simulink model "ADCS_trainee0"  (R2020b)
settings: Solver=ode23t  StartTime=0.0  StopTime=250  RelTol=1e-4
values from neighbouring files (symbols this model uses):
  J = eye(3)*((massa_sat*((d^2)/6))+Jr)    [ADCS_main_trainee.m]
  Jr = 3e-6    (= 3e-06)    [ADCS_main_trainee.m]
  mag_ref = [2 -5 3]'    [ADCS_main_trainee.m]
  sol_ref = [5 -1 1]'    [ADCS_main_trainee.m]
  T = 5    [ADCS_main_trainee.m]
  vel_ang_inicial = [0 6e-2 0]'    [ADCS_main_trainee.m]
undefined symbols (not defined in the file or in its folder): b, Kiw, Km, Kpw
libraries: vrlib x4, aerolibutil x3, pid_lib x2, aerolibanim x1, sharedutil x1, sharedtransform x1
settings Model: Creator=felip  LastModifiedBy=elder
settings SolverCC: ZeroCrossAlgorithm=Adaptive  AutoInsertRateTranBlk=on
settings DebuggingCC: IgnoredZcDiagnostic=none

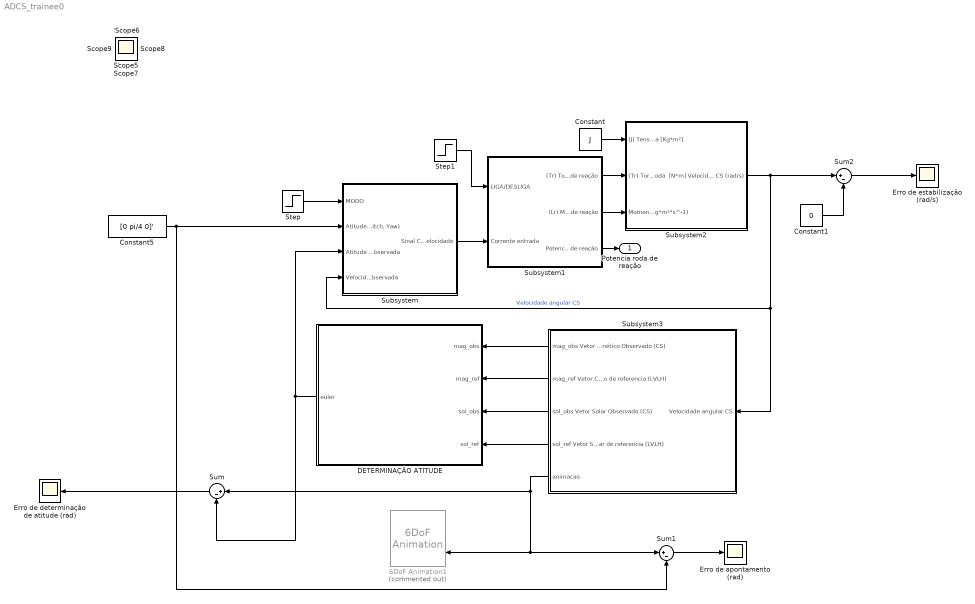
== system ADCS_trainee0 ==
  6DoF Animation1 : aerolibanim/6DoF Animation  Commented=on  u1=[-15 15 -15 15 -15 15]  u2=0.1  u3=0.81  u4=[0 0 0]  u5=Fly alongside  u6=[150 150 -150]  u7=10  u8=on
  Constant : Constant  Value=J
  Constant1 : Constant  Value=0
  Constant5 : Constant  Value=[0 pi/4 0]'
  DETERMINAÇÂO ATITUDE : MATLAB Function  TreatAsAtomicUnit=on  SystemSampleTime=1e-1
  Erro de apontamento (rad) : Scope
  Erro de determinação de atitude (rad) : Scope
  Erro de estabilização (rad/s) : Scope
  Step : Step  Time=130  Before=1  After=0  SampleTime=0
  Step1 : Step  Time=10  SampleTime=0
  Subsystem : Subsystem
      mask Display:
      | image('$imagefile'); % Use "Edit Image" on toolstrip to change.
      | 
      | port_label('input', 1, 'modo', 'texmode', 'on')
      | port_label('input', 2, 'ati_{des}', 'texmode', 'on')
      | port_label('input', 3, 'ati_{obs}', 'texmode', 'on')
      | port_label('input', 4, '\omega_{cs}', 'texmode', 'on')
      | 
      | port_label('output', 1, 'W_{ref}', 'texmode', 'on')
  Subsystem1 : Subsystem
      mask Display:
      | image('$imagefile'); % Use "Edit Image" on toolstrip to change.
      | port_label('input', 1, 'LIG/DES', 'texmode', 'on')
      | port_label('input', 2, 'W_{rr}', 'texmode', 'on')
      | 
      | port_label('output', 1, '\tau_{rr}', 'texmode', 'on')
      | port_label('output', 2, 'L_{rr}', 'texmode', 'on')
      | port_label('output', 3, 'P_{rr}', 'texmode', 'on')
  Subsystem2 : Subsystem
      mask Display:
      | image('$imagefile'); % Use "Edit Image" on toolstrip to change.
      | 
      | port_label('input', 1, 'J_{cs}', 'texmode', 'on')
      | port_label('input', 2, '\tau_{rr}', 'texmode', 'on')
      | port_label('input', 3, 'L_{rr}', 'texmode', 'on')
      | 
      | port_label('output', 1, '\omega_{cs}', 'texmode', 'on')
  Subsystem3 : Subsystem
      mask Display:
      | image('$imagefile'); % Use "Edit Image" on toolstrip to change.
      | 
      | port_label('input', 1, '\omega_{cs}', 'texmode', 'on')
      | 
      | 
      | port_label('output', 1, 'mag_{obs}', 'texmode', 'on')
      | port_label('output', 2, 'mag_{ref}', 'texmode', 'on')
      | port_label('output', 3, 'sol_{obs}', 'texmode', 'on')
      | port_label('output', 4, 'sol_{ref}', 'texmode', 'on')
      | port_label('output', 5, 'ati_{real}', 'texmode', 'on')
  Sum : Sum  Inputs=|+-
  Sum1 : Sum  Inputs=|+-
  Sum2 : Sum  Inputs=|+-
  Potencia roda de reação : Outport
  Scope{,1..9} (10 alike) : Scope
  wires:
  Step/1 -> Subsystem/1(MODO)
  Step1/1 -> Subsystem1/1(LIGA/DESLIGA)
  Subsystem/1(Sinal Controle Velocidade) -> Subsystem1/2(Corrente entrada)
  Constant/1 -> Subsystem2/1((J) Tensor de Inercia Satélite + roda [Kg*m²])
  Subsystem1/1((Tr) Torque roda de reação) -> Subsystem2/2((Tr) Torque roda  [N*m])
  Subsystem2/1(Velocidade angular CS (rad/s)) -> Sum2/1, Subsystem3/1(Velocidade angular CS), Subsystem/4(Velocidade angular CS observada)  "Velocidade angular CS"
  Subsystem3/1(mag_obs Vetor Campo magnético Observado (CS)) -> DETERMINAÇÂO ATITUDE/1(mag_obs)
  Subsystem3/2("mag_ref Vetor Campo magnético de referencia (LVLH) ") -> DETERMINAÇÂO ATITUDE/2(mag_ref)
  Subsystem3/3(sol_obs Vetor Solar Observado (CS)) -> DETERMINAÇÂO ATITUDE/3(sol_obs)
  Subsystem3/4(sol_ref Vetor Solar de referencia (LVLH)) -> DETERMINAÇÂO ATITUDE/4(sol_ref)
  Subsystem1/2((Lr) Momento angular roda de reação) -> Subsystem2/3(Momento angular roda  (kg*m²*s^-1))
  Constant5/1 -> Subsystem/2("Atitude desejada (Roll, Pitch, Yaw)"), Sum1/2
  Subsystem3/5(animacao) -> Sum1/1, 6DoF Animation1/2, Sum/1
  DETERMINAÇÂO ATITUDE/1(euler) -> Sum/2, Subsystem/3(Atitude observada)
  Sum/1 -> Erro de determinação de atitude (rad)/1
  Subsystem1/3(Potencia roda de reação) -> Potencia roda de reação/1
  Sum1/1 -> Erro de apontamento (rad)/1
  Sum2/1 -> Erro de estabilização (rad/s)/1
  Constant1/1 -> Sum2/2

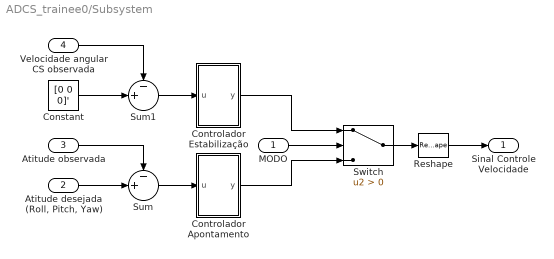
== system ADCS_trainee0/Subsystem ==
  MODO : Inport
  "Atitude desejada (Roll, Pitch, Yaw)" : Inport  Port=2
  Atitude observada : Inport  Port=3
  Velocidade angular CS observada : Inport  Port=4
  Constant : Constant  Value=[0 0 0]'
  Controlador Apontamento : Subsystem
      mask Display: set_param(gcb,'BackgroundColor','cyan')
  Controlador Estabilização : Subsystem
      mask Display: set_param(gcb,'BackgroundColor','cyan')
  Reshape : Reshape  OutputDimensionality=Column vector (2-D)
  Sum : Sum  Inputs=-+|
  Sum1 : Sum  Inputs=-+|
  Switch : Switch  Criteria=u2 > Threshold
  Sinal Controle Velocidade : Outport
  wires:
  MODO/1 -> Switch/2
  "Atitude desejada (Roll, Pitch, Yaw)"/1 -> Sum/2
  Switch/1 -> Reshape/1
  Reshape/1 -> Sinal Controle Velocidade/1
  Constant/1 -> Sum1/2
  Atitude observada/1 -> Sum/1
  Velocidade angular CS observada/1 -> Sum1/1
  Sum1/1 -> Controlador Estabilização/1(u)
  Controlador Estabilização/1(y) -> Switch/1
  Sum/1 -> Controlador Apontamento/1(u)
  Controlador Apontamento/1(y) -> Switch/3

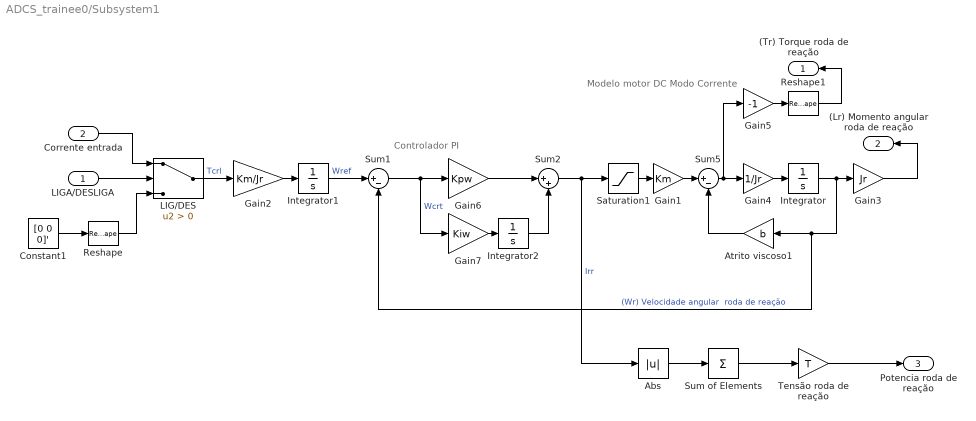
== system ADCS_trainee0/Subsystem1 ==
  note: Modelo motor DC
      | Modo Corrente
  note: Controlador PI
  LIGA/DESLIGA : Inport
  Corrente entrada : Inport  Port=2
  Abs : Abs
  Atrito viscoso1 : Gain  Gain=b
  Constant1 : Constant  Value=[0 0 0]'
  Gain1 : Gain  Gain=Km
  Gain2 : Gain  Gain=Km/Jr
  Gain3 : Gain  Gain=Jr
  Gain4 : Gain  Gain=1/Jr
  Gain5 : Gain  Gain=-1
  Gain6 : Gain  Gain=Kpw
  Gain7 : Gain  Gain=Kiw
  Integrator : Integrator
  Integrator1 : Integrator
  Integrator2 : Integrator
  LIG/DES : Switch  Criteria=u2 > Threshold
  Reshape : Reshape  OutputDimensionality=Column vector (2-D)
  Reshape1 : Reshape  OutputDimensionality=Column vector (2-D)
  Saturation1 : Saturate  ZeroCross=off
  Sum of Elements : Sum  Inputs=+
  Sum1 : Sum  Inputs=|+-
  Sum2 : Sum  Inputs=|++
  Sum5 : Sum  Inputs=|+-
  Tensão roda de reação : Gain  Gain=T
  (Tr) Torque roda de reação : Outport
  (Lr) Momento angular roda de reação : Outport  Port=2
  Potencia roda de reação : Outport  Port=3
  wires:
  Gain5/1 -> Reshape1/1
  Gain4/1 -> Integrator/1
  Constant1/1 -> Reshape/1
  Reshape/1 -> LIG/DES/3
  Gain1/1 -> Sum5/1
  Gain3/1 -> (Lr) Momento angular roda de reação/1
  Corrente entrada/1 -> LIG/DES/1
  Sum5/1 -> Gain5/1, Gain4/1
  Reshape1/1 -> (Tr) Torque roda de reação/1
  Integrator/1 -> Gain3/1, Sum1/2, Atrito viscoso1/1  "(Wr) Velocidade angular  roda de reação"
  LIGA/DESLIGA/1 -> LIG/DES/2
  Atrito viscoso1/1 -> Sum5/2
  Saturation1/1 -> Gain1/1
  LIG/DES/1 -> Gain2/1  "Tcrl"
  Gain2/1 -> Integrator1/1
  Integrator1/1 -> Sum1/1  "Wref"
  Gain7/1 -> Integrator2/1
  Sum1/1 -> Gain7/1, Gain6/1  "Wcrt"
  Gain6/1 -> Sum2/1
  Integrator2/1 -> Sum2/2
  Sum2/1 -> Abs/1, Saturation1/1  "Irr"
  Tensão roda de reação/1 -> Potencia roda de reação/1
  Sum of Elements/1 -> Tensão roda de reação/1
  Abs/1 -> Sum of Elements/1

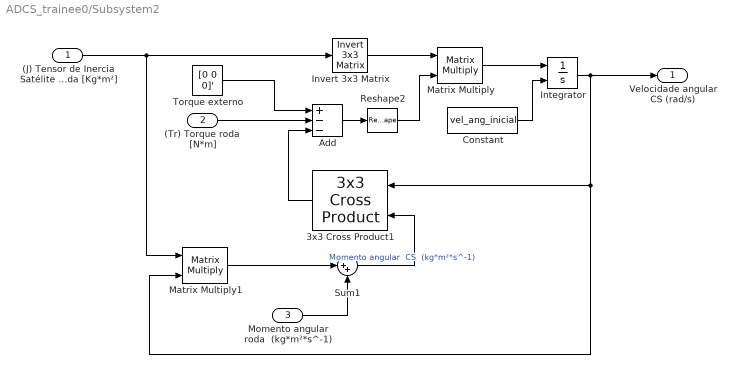
== system ADCS_trainee0/Subsystem2 ==
  (J) Tensor de Inercia Satélite + roda [Kg*m²] : Inport
  (Tr) Torque roda  [N*m] : Inport  Port=2  Unit=(kg*m*m)/s
  Momento angular roda  (kg*m²*s^-1) : Inport  Port=3  Unit=(kg*m*m)/s
  3x3 Cross Product1 : sharedutil/3x3 Cross Product  aMode=aMode
      settings: SourceProductBaseCode=AE,PW,MT,UV,VE,VP
  Add : Sum  Inputs=+--
  Constant : Constant  Value=vel_ang_inicial
  Integrator : Integrator  InitialConditionSource=external
  Invert 3x3 Matrix : aerolibutil/Invert  3x3 Matrix
  Matrix Multiply : Product  Multiplication=Matrix(*)
  Matrix Multiply1 : Product  Multiplication=Matrix(*)
  Reshape2 : Reshape  OutputDimensionality=Column vector (2-D)
  Sum1 : Sum  Inputs=|++
  Torque externo : Constant  Value=[0 0 0]'
  Velocidade angular CS (rad/s) : Outport
  wires:
  (Tr) Torque roda  [N*m]/1 -> Add/2
  (J) Tensor de Inercia Satélite + roda [Kg*m²]/1 -> Invert 3x3 Matrix/1, Matrix Multiply1/1
  Integrator/1 -> Velocidade angular CS (rad/s)/1, Matrix Multiply1/2, 3x3 Cross Product1/1
  Momento angular roda  (kg*m²*s^-1)/1 -> Sum1/2
  Matrix Multiply1/1 -> Sum1/1
  Torque externo/1 -> Add/1
  Reshape2/1 -> Matrix Multiply/2
  Constant/1 -> Integrator/2
  Add/1 -> Reshape2/1
  Matrix Multiply/1 -> Integrator/1
  Invert 3x3 Matrix/1 -> Matrix Multiply/1
  Sum1/1 -> 3x3 Cross Product1/2  "Momento angular  CS  (kg*m²*s^-1)"
  3x3 Cross Product1/1 -> Add/3

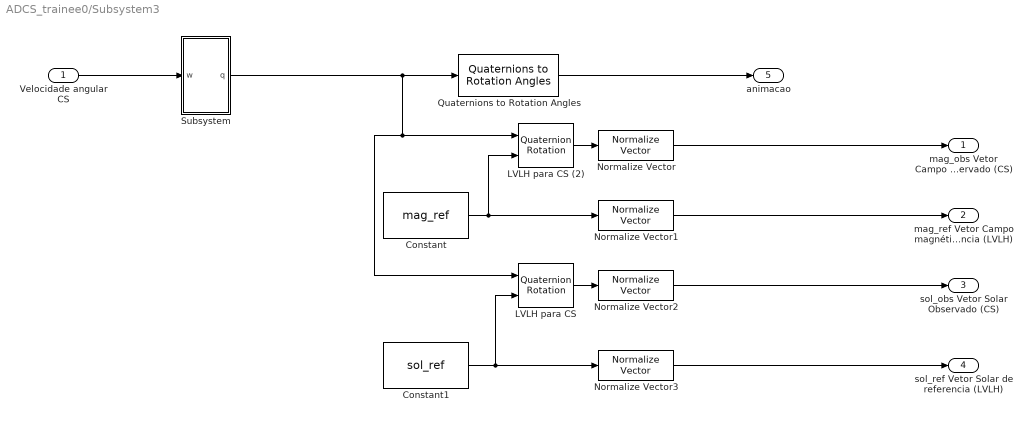
== system ADCS_trainee0/Subsystem3 ==
  Velocidade angular CS : Inport
  Constant : Constant  Value=mag_ref
  Constant1 : Constant  Value=sol_ref
  LVLH para CS : aerolibutil/Quaternion Rotation
  LVLH para CS (2) : aerolibutil/Quaternion Rotation
  Normalize Vector{,1..3} (4 alike) : vrlib/Utilities/Normalize Vector  maxzero=0
  Quaternions to Rotation Angles : sharedtransform/Quaternions to Rotation Angles  rotationOrder=XYZ  aMode=aMode
      settings: SourceProductBaseCode=AE,PW,MT,UV,VE,VP
  Subsystem : Subsystem
  mag_obs Vetor Campo magnético Observado (CS) : Outport
  "mag_ref Vetor Campo magnético de referencia (LVLH) " : Outport  Port=2
  sol_obs Vetor Solar Observado (CS) : Outport  Port=3
  sol_ref Vetor Solar de referencia (LVLH) : Outport  Port=4
  animacao : Outport  Port=5
  wires:
  LVLH para CS/1 -> Normalize Vector2/1
  Constant/1 -> Normalize Vector1/1, LVLH para CS (2)/2
  Constant1/1 -> LVLH para CS/2, Normalize Vector3/1
  Normalize Vector/1 -> mag_obs Vetor Campo magnético Observado (CS)/1
  Quaternions to Rotation Angles/1 -> animacao/1
  LVLH para CS (2)/1 -> Normalize Vector/1
  Normalize Vector1/1 -> "mag_ref Vetor Campo magnético de referencia (LVLH) "/1
  Normalize Vector2/1 -> sol_obs Vetor Solar Observado (CS)/1
  Normalize Vector3/1 -> sol_ref Vetor Solar de referencia (LVLH)/1
  Subsystem/1(q) -> Quaternions to Rotation Angles/1, LVLH para CS (2)/1, LVLH para CS/1
  Velocidade angular CS/1 -> Subsystem/1(w)

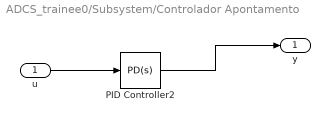
== system ADCS_trainee0/Subsystem/Controlador Apontamento ==
  u : Inport
  PID Controller2 : pid_lib/PID Controller  Controller=PD  Form=Parallel  TimeDomain=Continuous-time  UseExternalTs=off  SampleTime=-1  IntegratorMethod=Forward Euler  FilterMethod=Forward Euler  ControllerParametersSource=internal  P=0.04  I=100  D=0.2  UseFilter=on  N=5  TunerSelectOption=Transfer Function Based (PID Tuner App)  ZeroCross=off  InitialConditionSource=internal  InitialConditionForIntegrator=0  InitialConditionForFilter=0  DifferentiatorICPrevScaledInput=0  ExternalReset=none  TrackingMode=off  Kt=1  LimitOutput=off  SatLimitsSource=internal  UpperSaturationLimit=inf  LowerSaturationLimit=-inf  LinearizeAsGain=on  AntiWindupMode=none  Kb=1  PGainOutDataTypeStr=double  PProdOutDataTypeStr=double  POutMin=[]  POutMax=[]  IOutMin=[]  IOutMax=[]  DGainOutDataTypeStr=double  DProdOutDataTypeStr=double  DOutMin=[]  DOutMax=[]  NGainOutDataTypeStr=double  NProdOutDataTypeStr=double  NOutMin=[]  NOutMax=[]  SumOutDataTypeStr=double  SumOutMin=[]  SumOutMax=[]  SaturationOutMin=[]  SaturationOutMax=[]  PParamMin=[]  PParamMax=[]  IParamMin=[]  IParamMax=[]  DParamMin=[]  DParamMax=[]  NParamMin=[]  NParamMax=[]  KbParamMin=[]  KbParamMax=[]  KtParamMin=[]  KtParamMax=[]  KbOutMin=[]  KbOutMax=[]  KtOutMin=[]  KtOutMax=[]  IntegratorOutMin=[]  IntegratorOutMax=[]  FilterOutMin=[]  FilterOutMax=[]  SumI1OutMin=[]  SumI1OutMax=[]  SumI2OutMin=[]  SumI2OutMax=[]  SumI3OutMin=[]  SumI3OutMax=[]  SumI4OutMin=[]  SumI4OutMax=[]  SumDOutMin=[]  SumDOutMax=[]  DifferentiatorOutMin=[]  DifferentiatorOutMax=[]  FilterDiffOutCoefMin=[]  FilterDiffOutCoefMax=[]  ReciprocalOutMin=[]  ReciprocalOutMax=[]  SumDenOutMin=[]  SumDenOutMax=[]  SumNumOutMin=[]  SumNumOutMax=[]  DivideOutMin=[]  DivideOutMax=[]  UdiffTsProdOutMin=[]  UdiffTsProdOutMax=[]  NTsProdOutMin=[]  NTsProdOutMax=[]  UintegralTsProdOutMin=[]  UintegralTsProdOutMax=[]  UngainTsProdOutMin=[]  UngainTsProdOutMax=[]  IntegratorContinuousStateAttributes=''  IntegratorStateMustResolveToSignalObject=off  IntegratorRTWStateStorageClass=Auto  FilterContinuousStateAttributes=''  FilterStateMustResolveToSignalObject=off  FilterRTWStateStorageClass=Auto  ParallelPVariant=InternalParameters  IdealPVariant=Disabled  IVariant=Disabled  DVariant=InternalParameters  IntegratorVariant=Disabled  SatVariant=Disabled  AWVariant=Disabled  PCopyVariant=Disabled  TRVariant=Disabled  FdbkBlocksVariant=Forward  IdealPFdbkVariant=Disabled  SatFdbkVariant=Disabled  DerivativeFilterVariant=ContFilter  NVariant=InternalParameters  NCopyVariant=Disabled  FilterICVariant=InternalICsFilter  IntegratorICVariant=Disabled  ExternalResetVariant=Disabled  TRSumVariant=Passthrough  SumFdbkVariant=Disabled  SumVariant=Sum_PD  TsampFilterVariant=InternalTs  TsampNgainVariant=Passthrough  TsampIntegralVariant=Disabled_SignalSpec  ExternalSaturationOutDataTypeStr=Inherit: Same as second input
  y : Outport
  wires:
  u/1 -> PID Controller2/1
  PID Controller2/1 -> y/1

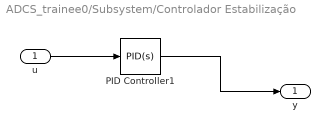
== system ADCS_trainee0/Subsystem/Controlador Estabilização ==
  u : Inport
  PID Controller1 : pid_lib/PID Controller  Controller=PID  Form=Parallel  TimeDomain=Continuous-time  UseExternalTs=off  SampleTime=-1  IntegratorMethod=Forward Euler  FilterMethod=Forward Euler  ControllerParametersSource=internal  P=0.8  I=0.2  D=0.75  UseFilter=on  N=100  TunerSelectOption=Transfer Function Based (PID Tuner App)  InitialConditionSource=internal  InitialConditionForIntegrator=0  InitialConditionForFilter=0  DifferentiatorICPrevScaledInput=0  ExternalReset=none  TrackingMode=off  Kt=1  LimitOutput=off  SatLimitsSource=internal  UpperSaturationLimit=inf  LowerSaturationLimit=-inf  LinearizeAsGain=on  AntiWindupMode=none  Kb=1  POutMin=[]  POutMax=[]  IOutMin=[]  IOutMax=[]  DOutMin=[]  DOutMax=[]  NOutMin=[]  NOutMax=[]  SumOutMin=[]  SumOutMax=[]  SaturationOutMin=[]  SaturationOutMax=[]  PParamMin=[]  PParamMax=[]  IParamMin=[]  IParamMax=[]  DParamMin=[]  DParamMax=[]  NParamMin=[]  NParamMax=[]  KbParamMin=[]  KbParamMax=[]  KtParamMin=[]  KtParamMax=[]  KbOutMin=[]  KbOutMax=[]  KtOutMin=[]  KtOutMax=[]  IntegratorOutMin=[]  IntegratorOutMax=[]  FilterOutMin=[]  FilterOutMax=[]  SumI1OutMin=[]  SumI1OutMax=[]  SumI2OutMin=[]  SumI2OutMax=[]  SumI3OutMin=[]  SumI3OutMax=[]  SumI4OutMin=[]  SumI4OutMax=[]  SumDOutMin=[]  SumDOutMax=[]  DifferentiatorOutMin=[]  DifferentiatorOutMax=[]  FilterDiffOutCoefMin=[]  FilterDiffOutCoefMax=[]  ReciprocalOutMin=[]  ReciprocalOutMax=[]  SumDenOutMin=[]  SumDenOutMax=[]  SumNumOutMin=[]  SumNumOutMax=[]  DivideOutMin=[]  DivideOutMax=[]  UdiffTsProdOutMin=[]  UdiffTsProdOutMax=[]  NTsProdOutMin=[]  NTsProdOutMax=[]  UintegralTsProdOutMin=[]  UintegralTsProdOutMax=[]  UngainTsProdOutMin=[]  UngainTsProdOutMax=[]  IntegratorContinuousStateAttributes=''  IntegratorStateMustResolveToSignalObject=off  IntegratorRTWStateStorageClass=Auto  FilterContinuousStateAttributes=''  FilterStateMustResolveToSignalObject=off  FilterRTWStateStorageClass=Auto  ParallelPVariant=InternalParameters  IdealPVariant=Disabled  IVariant=InternalParameters  DVariant=InternalParameters  IntegratorVariant=Continuous  SatVariant=Disabled  AWVariant=Passthrough  PCopyVariant=Disabled  TRVariant=Disabled  FdbkBlocksVariant=Forward  IdealPFdbkVariant=Disabled  SatFdbkVariant=Disabled  DerivativeFilterVariant=ContFilter  NVariant=InternalParameters  NCopyVariant=Disabled  FilterICVariant=InternalICsFilter  IntegratorICVariant=InternalICs  ExternalResetVariant=Disabled  TRSumVariant=Passthrough  SumFdbkVariant=Disabled  SumVariant=Sum_PID  TsampFilterVariant=InternalTs  TsampNgainVariant=Passthrough  TsampIntegralVariant=Passthrough  ExternalSaturationOutDataTypeStr=Inherit: Same as second input
  y : Outport
  wires:
  u/1 -> PID Controller1/1
  PID Controller1/1 -> y/1

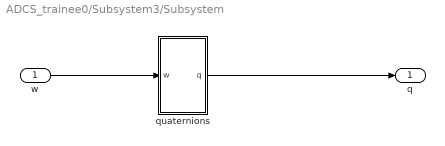
== system ADCS_trainee0/Subsystem3/Subsystem ==
  w : Inport
  quaternions : Subsystem
  q : Outport
  wires:
  quaternions/1(q) -> q/1
  w/1 -> quaternions/1(w)

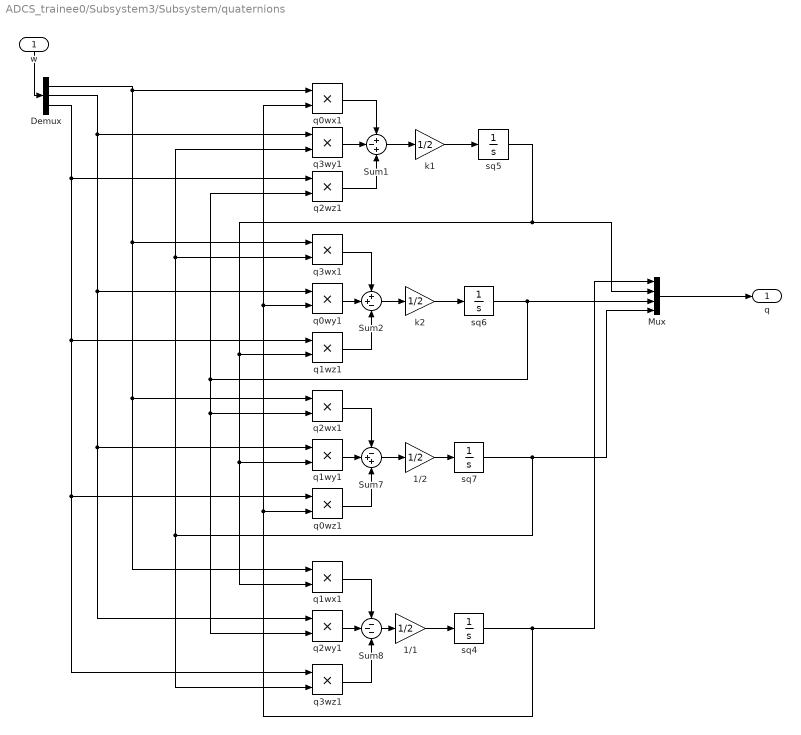
== system ADCS_trainee0/Subsystem3/Subsystem/quaternions ==
  w : Inport
  1/1 : Gain  Gain=1/2
  1/2 : Gain  Gain=1/2
  Demux : Demux  Outputs=3
  Mux : Mux
  Sum1 : Sum  Inputs=+-+
  Sum2 : Sum  Inputs=++-
  Sum7 : Sum  Inputs=-++
  Sum8 : Sum  Inputs=---
  k1 : Gain  Gain=1/2
  k2 : Gain  Gain=1/2
  q0wx1 : Product  RndMeth=Zero
  q0wy1 : Product  RndMeth=Zero
  q0wz1 : Product  RndMeth=Zero
  q1wx1 : Product  RndMeth=Zero
  q1wy1 : Product  RndMeth=Zero
  q1wz1 : Product  RndMeth=Zero
  q2wx1 : Product  RndMeth=Zero
  q2wy1 : Product  RndMeth=Zero
  q2wz1 : Product  RndMeth=Zero
  q3wx1 : Product  RndMeth=Zero
  q3wy1 : Product  RndMeth=Zero
  q3wz1 : Product  RndMeth=Zero
  sq4 : Integrator  InitialCondition=1
  sq5 : Integrator
  sq6 : Integrator
  sq7 : Integrator
  q : Outport
  wires:
  Sum8/1 -> 1/1/1
  q3wz1/1 -> Sum8/3
  k1/1 -> sq5/1
  1/1/1 -> sq4/1
  sq6/1 -> q2wy1/2, q2wx1/2, q2wz1/2, Mux/3
  q2wz1/1 -> Sum1/3
  sq7/1 -> q3wz1/2, q3wx1/2, q3wy1/2, Mux/4
  Sum7/1 -> 1/2/1
  sq5/1 -> q1wx1/2, q1wy1/2, q1wz1/2, Mux/2
  q2wx1/1 -> Sum7/1
  q1wx1/1 -> Sum8/1
  k2/1 -> sq6/1
  q0wy1/1 -> Sum2/2
  q1wy1/1 -> Sum7/2
  sq4/1 -> q0wz1/2, q0wy1/2, q0wx1/2, Mux/1
  1/2/1 -> sq7/1
  Demux/2 -> q2wy1/1, q1wy1/1, q0wy1/1, q3wy1/1
  q3wx1/1 -> Sum2/1
  q0wz1/1 -> Sum7/3
  q1wz1/1 -> Sum2/3
  Sum1/1 -> k1/1
  q0wx1/1 -> Sum1/1
  q3wy1/1 -> Sum1/2
  Demux/1 -> q1wx1/1, q2wx1/1, q3wx1/1, q0wx1/1
  Sum2/1 -> k2/1
  q2wy1/1 -> Sum8/2
  Demux/3 -> q3wz1/1, q0wz1/1, q1wz1/1, q2wz1/1
  Mux/1 -> q/1
  w/1 -> Demux/1

== matlab function ADCS_trainee0/DETERMINAÇÂO ATITUDE ==
  data: mag_obs input; mag_ref input; euler output; sol_obs input; sol_ref input
function euler = fcn(mag_obs,mag_ref,sol_obs,sol_ref)
%% Vetores t1, t2 e t3 para as medições no BFCS (Body Fixed Coordinate System)
% Considera-se que o sensor ? é o sensor mais preciso


%% Vetores t1, t2 e t3 para a referência no ECI (Earth Centered Inertial Frame)


%% Determinação das tríades S e R e da matriz de rotação A


%% Determinação dos ângulos de Euler


    euler = [phi; theta; psi];
